simulink model "PID"  (R2023a)
settings: Solver=VariableStepAuto  StartTime=0.0  StopTime=2.5  RelTol=1e-3
libraries: slpidlib x1
settings Model: Creator=Abdulrahman Hamdy  LastModifiedBy=Abderrahman

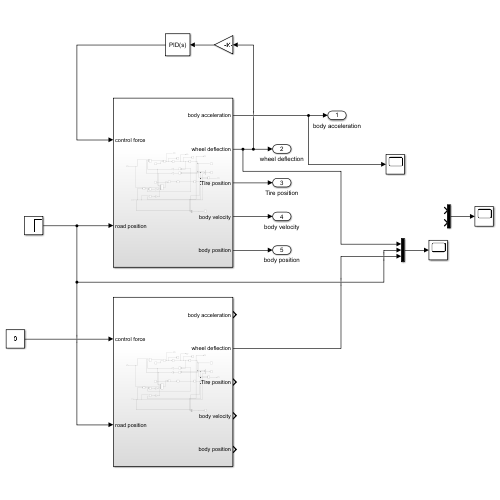
[thumbnail: Simulink's stored preview of the top-level diagram]
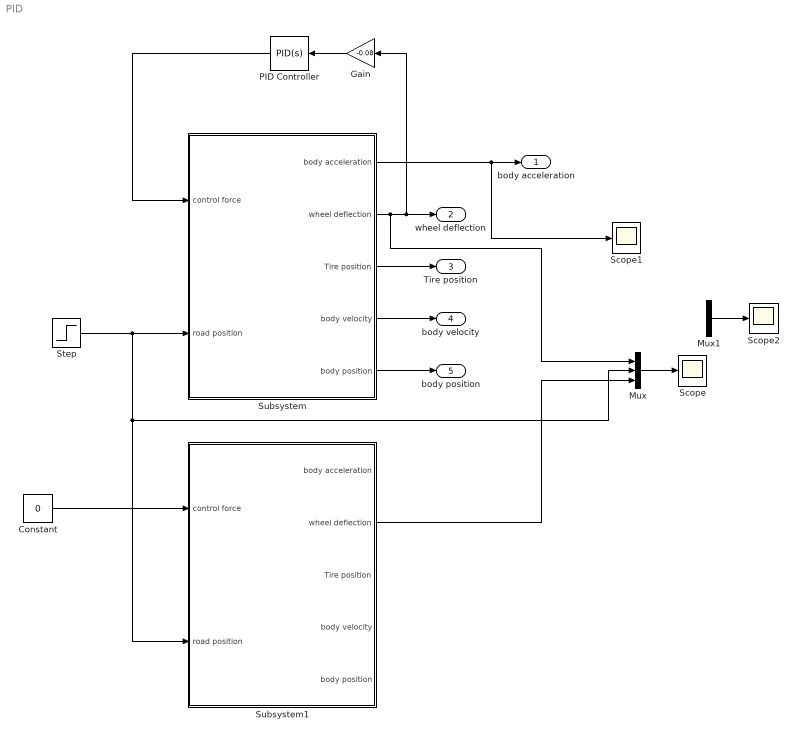
== system PID ==
  Constant : Constant  Value=0
  Gain : Gain  Gain=-0.08
  Mux : Mux  Inputs=3
  Mux1 : Mux  Inputs=2
  PID Controller : slpidlib/PID Controller  Controller=PID  Form=Parallel  TimeDomain=Continuous-time  UseExternalTs=off  SampleTime=-1  IntegratorMethod=Forward Euler  FilterMethod=Forward Euler  ControllerParametersSource=internal  P=8321  I=6240  UseKiTs=off  D=20802  N=1000  UseFilter=on  TunerSelectOption=Transfer Function Based (PID Tuner App)  InitialConditionSource=internal  InitialConditionForIntegrator=0  InitialConditionForFilter=0  DifferentiatorICPrevScaledInput=0  ExternalReset=none  TrackingMode=off  Kt=1  LimitOutput=off  SatLimitsSource=internal  UpperSaturationLimit=inf  LowerSaturationLimit=-inf  LinearizeAsGain=on  AntiWindupMode=none  Kb=1  LimitIntegrator=off  UpperIntegratorSaturationLimit=inf  LowerIntegratorSaturationLimit=-inf  POutMin=[]  POutMax=[]  IOutMin=[]  IOutMax=[]  DOutMin=[]  DOutMax=[]  NOutMin=[]  NOutMax=[]  SumOutMin=[]  SumOutMax=[]  SaturationOutMin=[]  SaturationOutMax=[]  PParamMin=[]  PParamMax=[]  IParamMin=[]  IParamMax=[]  DParamMin=[]  DParamMax=[]  NParamMin=[]  NParamMax=[]  KbParamMin=[]  KbParamMax=[]  KtParamMin=[]  KtParamMax=[]  KbOutMin=[]  KbOutMax=[]  KtOutMin=[]  KtOutMax=[]  IntegratorOutMin=[]  IntegratorOutMax=[]  FilterOutMin=[]  FilterOutMax=[]  SumI1OutMin=[]  SumI1OutMax=[]  SumI2OutMin=[]  SumI2OutMax=[]  SumI3OutMin=[]  SumI3OutMax=[]  SumI4OutMin=[]  SumI4OutMax=[]  SumDOutMin=[]  SumDOutMax=[]  DifferentiatorOutMin=[]  DifferentiatorOutMax=[]  FilterDiffOutCoefMin=[]  FilterDiffOutCoefMax=[]  ReciprocalOutMin=[]  ReciprocalOutMax=[]  SumDenOutMin=[]  SumDenOutMax=[]  SumNumOutMin=[]  SumNumOutMax=[]  DivideOutMin=[]  DivideOutMax=[]  UdiffTsProdOutMin=[]  UdiffTsProdOutMax=[]  NTsProdOutMin=[]  NTsProdOutMax=[]  UintegralTsProdOutMin=[]  UintegralTsProdOutMax=[]  UngainTsProdOutMin=[]  UngainTsProdOutMax=[]  ClampingZeroOutDataTypeStr=Inherit: Inherit via back propagation  ClampingZeroOutMin=[]  ClampingZeroOutMax=[]  FilterDenConstantOutDataTypeStr=Inherit: Inherit via back propagation  FilterDenConstantOutMin=[]  FilterDenConstantOutMax=[]  PCopyOutDataTypeStr=Inherit: Inherit via back propagation  PCopyOutMin=[]  PCopyOutMax=[]  NCopyOutDataTypeStr=Inherit: Inherit via back propagation  NCopyOutMin=[]  NCopyOutMax=[]  IntegratorContinuousStateAttributes=''  IntegratorStateMustResolveToSignalObject=off  IntegratorRTWStateStorageClass=Auto  FilterContinuousStateAttributes=''  FilterStateMustResolveToSignalObject=off  FilterRTWStateStorageClass=Auto  ParallelPVariant=InternalParameters  IdealPVariant=Disabled  IVariant=InternalParameters  DVariant=InternalParameters  IntegratorVariant=Continuous  SatVariant=Disabled  AWVariant=Passthrough  PCopyVariant=Disabled  TRVariant=Disabled  FdbkBlocksVariant=Forward  IdealPFdbkVariant=Disabled  SatFdbkVariant=Disabled  DerivativeFilterVariant=ContFilter  NVariant=InternalParameters  NCopyVariant=Disabled  FilterICVariant=InternalICsFilter  IntegratorICVariant=InternalICs  ExternalResetVariant=Disabled  TRSumVariant=Passthrough  SumFdbkVariant=Disabled  SumVariant=Sum_PID  TsampFilterVariant=InternalTs  TsampNgainVariant=Passthrough  TsampIntegralVariant=Disabled_SignalSpec  ExternalSaturationOutDataTypeStr=Inherit: Same as second input
  Scope : Scope
  Scope1 : Scope
  Scope2 : Scope
  Step : Step  Time=0  SampleTime=0
  Subsystem : Subsystem
  Subsystem1 : Subsystem
  body acceleration : Outport
  wheel deflection : Outport  Port=2
  Tire position : Outport  Port=3
  body velocity : Outport  Port=4
  body position : Outport  Port=5
  wires:
  Subsystem/2(wheel deflection) -> Mux/1, Gain/1, wheel deflection/1
  Subsystem/3(Tire position) -> Tire position/1
  Subsystem/4(body velocity) -> body velocity/1
  Subsystem/5(body position) -> body position/1
  Mux/1 -> Scope/1
  Subsystem/1(body acceleration) -> Scope1/1, body acceleration/1
  Step/1 -> Subsystem1/2(road position), Mux/2, Subsystem/2(road position)
  PID Controller/1 -> Subsystem/1(control force)
  Gain/1 -> PID Controller/1
  Constant/1 -> Subsystem1/1(control force)
  Mux1/1 -> Scope2/1
  Subsystem1/2(wheel deflection) -> Mux/3

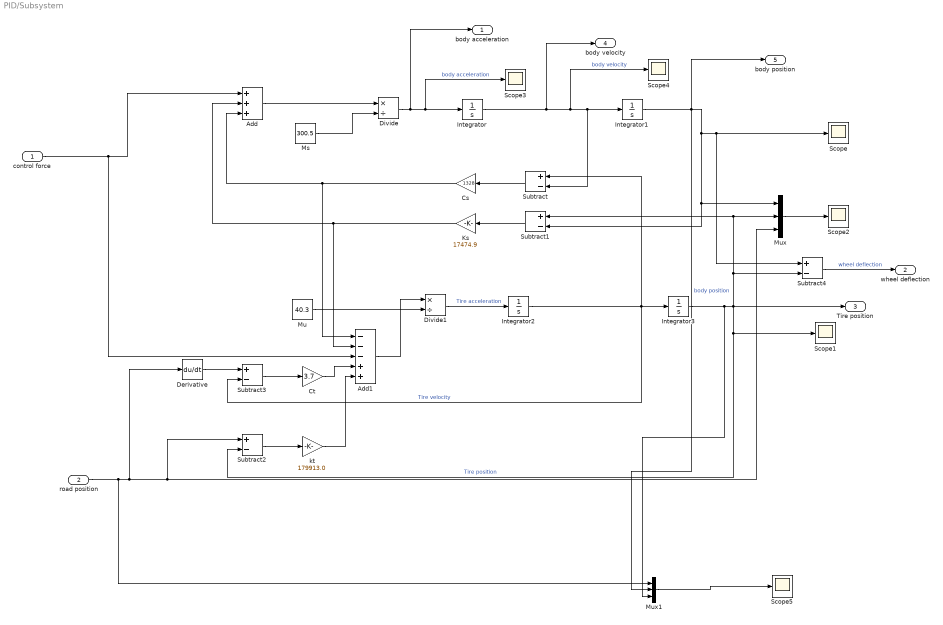
== system PID/Subsystem ==
  control force : Inport
  road position : Inport  Port=2
  Add : Sum  Inputs=+++
  Add1 : Sum  Inputs=---++
  Cs : Gain  Gain=1328
  Ct : Gain  Gain=3.7
  Derivative : Derivative
  Divide : Product  Inputs=*/
  Divide1 : Product  Inputs=*/
  Integrator{,1..3} (4 alike) : Integrator
  Ks : Gain  Gain=17474.9
  Ms : Constant  Value=300.5
  Mu : Constant  Value=40.3
  Mux : Mux  Inputs=3
  Mux1 : Mux  Inputs=3
  Scope{,1..5} (6 alike) : Scope
  Subtract{,1..4} (5 alike) : Sum  Inputs=+-
  kt : Gain  Gain=179913.0
  body acceleration : Outport
  wheel deflection : Outport  Port=2
  Tire position : Outport  Port=3
  body velocity : Outport  Port=4
  body position : Outport  Port=5
  wires:
  Ms/1 -> Divide/2
  Integrator1/1 -> body position/1, Mux1/2, Mux/1, Subtract1/2, Scope/1, Subtract4/1  "body position"
  Integrator2/1 -> Subtract/1, Subtract3/2, Integrator3/1  "Tire velocity"
  Integrator3/1 -> Mux1/3, Tire position/1, Subtract4/2, Mux/2, Subtract1/1, Scope1/1, Subtract2/2  "Tire position"
  Ks/1 -> Add1/2, Add/2
  Ct/1 -> Add1/4
  Integrator/1 -> body velocity/1, Scope4/1, Subtract/2, Integrator1/1  "body velocity"
  road position/1 -> Mux1/1, Derivative/1, Subtract2/1, Mux/3
  Subtract3/1 -> Ct/1
  control force/1 -> Add1/3, Add/1
  Divide/1 -> body acceleration/1, Scope3/1, Integrator/1  "body acceleration"
  Cs/1 -> Add1/1, Add/3
  Add1/1 -> Divide1/1
  Add/1 -> Divide/1
  kt/1 -> Add1/5
  Mu/1 -> Divide1/2
  Divide1/1 -> Integrator2/1  "Tire acceleration"
  Derivative/1 -> Subtract3/1
  Mux1/1 -> Scope5/1
  Subtract1/1 -> Ks/1
  Subtract/1 -> Cs/1
  Mux/1 -> Scope2/1
  Subtract2/1 -> kt/1
  Subtract4/1 -> wheel deflection/1  "wheel deflection"

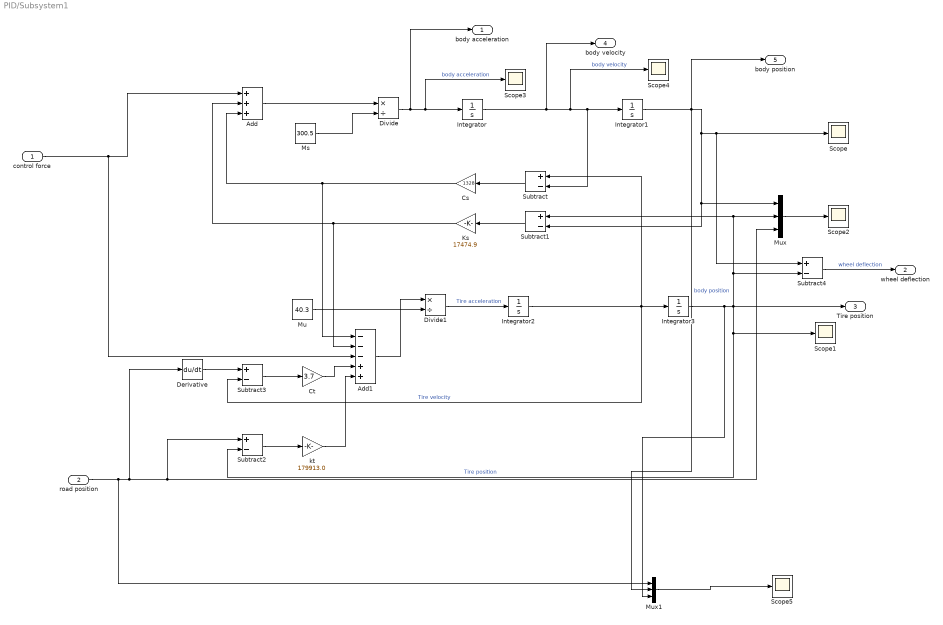
== system PID/Subsystem1 ==
  control force : Inport
  road position : Inport  Port=2
  Add : Sum  Inputs=+++
  Add1 : Sum  Inputs=---++
  Cs : Gain  Gain=1328
  Ct : Gain  Gain=3.7
  Derivative : Derivative
  Divide : Product  Inputs=*/
  Divide1 : Product  Inputs=*/
  Integrator{,1..3} (4 alike) : Integrator
  Ks : Gain  Gain=17474.9
  Ms : Constant  Value=300.5
  Mu : Constant  Value=40.3
  Mux : Mux  Inputs=3
  Mux1 : Mux  Inputs=3
  Scope{,1..5} (6 alike) : Scope
  Subtract{,1..4} (5 alike) : Sum  Inputs=+-
  kt : Gain  Gain=179913.0
  body acceleration : Outport
  wheel deflection : Outport  Port=2
  Tire position : Outport  Port=3
  body velocity : Outport  Port=4
  body position : Outport  Port=5
  wires:
  Ms/1 -> Divide/2
  Integrator1/1 -> body position/1, Mux1/2, Mux/1, Subtract1/2, Scope/1, Subtract4/1  "body position"
  Integrator2/1 -> Subtract/1, Subtract3/2, Integrator3/1  "Tire velocity"
  Integrator3/1 -> Mux1/3, Tire position/1, Subtract4/2, Mux/2, Subtract1/1, Scope1/1, Subtract2/2  "Tire position"
  Ks/1 -> Add1/2, Add/2
  Ct/1 -> Add1/4
  Integrator/1 -> body velocity/1, Scope4/1, Subtract/2, Integrator1/1  "body velocity"
  road position/1 -> Mux1/1, Derivative/1, Subtract2/1, Mux/3
  Subtract3/1 -> Ct/1
  control force/1 -> Add1/3, Add/1
  Divide/1 -> body acceleration/1, Scope3/1, Integrator/1  "body acceleration"
  Cs/1 -> Add1/1, Add/3
  Add1/1 -> Divide1/1
  Add/1 -> Divide/1
  kt/1 -> Add1/5
  Mu/1 -> Divide1/2
  Divide1/1 -> Integrator2/1  "Tire acceleration"
  Derivative/1 -> Subtract3/1
  Mux1/1 -> Scope5/1
  Subtract1/1 -> Ks/1
  Subtract/1 -> Cs/1
  Mux/1 -> Scope2/1
  Subtract2/1 -> kt/1
  Subtract4/1 -> wheel deflection/1  "wheel deflection"
